simulink model "SIMULINK_ADP_Tracking"  (R2023b)
settings: Solver=FixedStepAuto  StartTime=0.0  StopTime=sim_end_time  FixedStep=fixed_step_size  RelTol=1e-3
undefined symbols (not defined in the file): a, act_end, b, battery_threshold, bb, delta_, draw_gif, droneyeeUAV2_NUM, droneyeeUAV3_NUM, droneyeeUAV4_NUM, droneyeeUAV5_NUM, fixed_step_size, k, KD_x, KD_y, kd_z, KDD_x, KDD_y, KI_x, KI_y, ki_z, KII_x, KII_y, KP_x, KP_y, kp_z, KPP_x, KPP_y, lmt, omega, omega_, R, sim_end_time, uav10num, uav1num, uav2num, uav3num, uav4num, uav5num, uav6num, uav7num, uav8num, uav9num, UAV_NUM, Vel_Switch_1, Vel_Switch_10, Vel_Switch_11, Vel_Switch_12, Vel_Switch_13, Vel_Switch_14, Vel_Switch_15, Vel_Switch_16, Vel_Switch_17, Vel_Switch_18, Vel_Switch_19, Vel_Switch_2, Vel_Switch_20, Vel_Switch_3, Vel_Switch_4, Vel_Switch_5 ... (+16)
libraries: simulink x118, aerolibanimutils x1
(part 3 of 11)

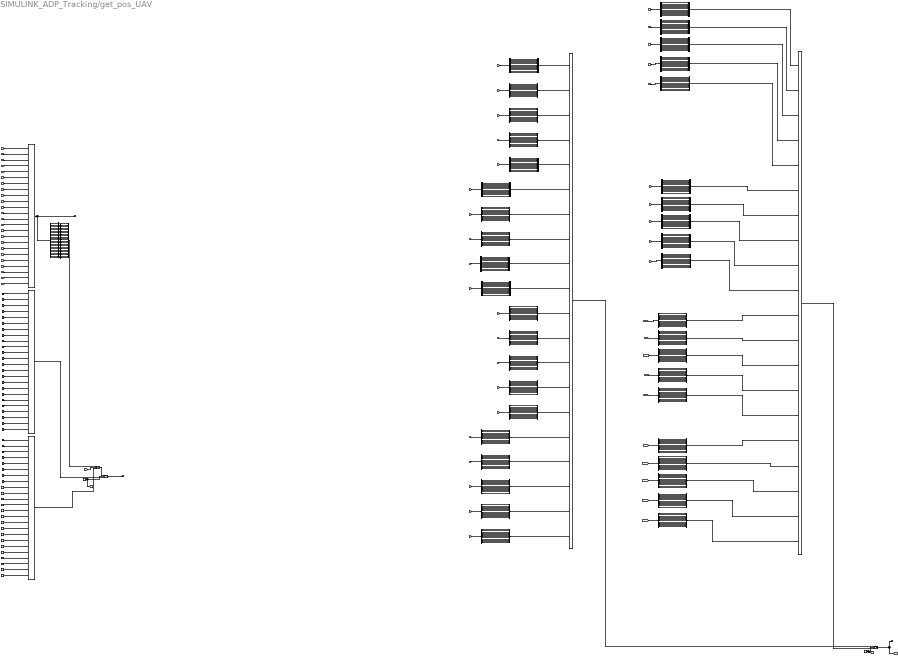
== system SIMULINK_ADP_Tracking/get_pos_UAV ==
  Bus Creator{1..20,37..42,46..49,51..60} (40 alike) : BusCreator  Inputs=12
  Bus Creator{34..36,62} (4 alike) : BusCreator  Inputs=24
  Bus Creator50 : BusCreator  Inputs=20
  Bus Creator61 : BusCreator  Inputs=20
  Bus Selector : BusSelector  OutputSignals=droneyeeUAV1bat,droneyeeUAV2bat,droneyeeUAV3bat,droneyeeUAV4bat,droneyeeUAV5bat,droneyeeUAV6bat,droneyeeUAV7bat,droneyeeUAV8bat,droneyeeUAV9bat,droneyeeUAV10bat,droneyeeUAV11bat,droneyeeUAV12bat,droneyeeUAV13bat,droneyeeUAV14bat,droneyeeUAV15bat,droneyeeUAV16bat,droneyeeUAV17bat,droneyeeUAV18bat,droneyeeUAV19bat,droneyeeUAV20bat,droneyeeUAV21bat,droneyeeUAV22bat,droneyeeUAV23bat,droneyeeUAV24bat
  Constant{,1..24} (25 alike) : Constant  Value=-1
  Constant25 : Constant
  Constant{26..49} (24 alike) : Constant  Value=100
  Demux{,16..23,40..41,52..57,59..62,66,68..69} (24 alike) : Demux  Outputs=3
  Demux{1..15,24..29,70..71,74..90} (40 alike) : Demux  Outputs=12
  Switch : Switch  SaturateOnIntegerOverflow=off  InputSameDT=off
  Switch1 : Switch  Criteria=u2 > Threshold  OutDataTypeStr=Inherit: Inherit via back propagation  SaturateOnIntegerOverflow=off  InputSameDT=off
  Switch2 : Switch  Criteria=u2 > Threshold  OutDataTypeStr=Inherit: Inherit via back propagation  SaturateOnIntegerOverflow=off  InputSameDT=off
  droneyeeUAV_batDIS : Outport  VectorParamsAs1DForOutWhenUnconnected=off
  droneyeeUAVbat1 : Outport  Port=2  VectorParamsAs1DForOutWhenUnconnected=off
  states1 : Outport  Port=3  VectorParamsAs1DForOutWhenUnconnected=off
  tag scope: sim_flag=global, switch_flag=global, uav_states=global
  wires:
  [battery_3] -> Bus Creator35/3  "droneyeeUAV3bat"
  [battery_1] -> Bus Creator35/1  "droneyeeUAV1bat"
  [battery_9] -> Bus Creator35/9  "droneyeeUAV9bat"
  [battery_2] -> Bus Creator35/2  "droneyeeUAV2bat"
  [battery_17] -> Bus Creator35/17  "droneyeeUAV17bat"
  [battery_6] -> Bus Creator35/6  "droneyeeUAV6bat"
  [battery_15] -> Bus Creator35/15  "droneyeeUAV15bat"
  [battery_12] -> Bus Creator35/12  "droneyeeUAV12bat"
  [battery_16] -> Bus Creator35/16  "droneyeeUAV16bat"
  [battery_11] -> Bus Creator35/11  "droneyeeUAV11bat"
  [battery_13] -> Bus Creator35/13  "droneyeeUAV13bat"
  [battery_19] -> Bus Creator35/19  "droneyeeUAV19bat"
  [battery_14] -> Bus Creator35/14  "droneyeeUAV14bat"
  [battery_20] -> Bus Creator35/20  "droneyeeUAV20bat"
  [battery_10] -> Bus Creator35/10  "droneyeeUAV10bat"
  Bus Creator35/1 -> Bus Selector/1, droneyeeUAV_batDIS/1
  [battery_18] -> Bus Creator35/18  "droneyeeUAV18bat"
  [battery_7] -> Bus Creator35/7  "droneyeeUAV7bat"
  [battery_8] -> Bus Creator35/8  "droneyeeUAV8bat"
  [battery_4] -> Bus Creator35/4  "droneyeeUAV4bat"
  [battery_23] -> Bus Creator35/23  "droneyeeUAV23bat"
  [battery_22] -> Bus Creator35/22  "droneyeeUAV22bat"
  [battery_21] -> Bus Creator35/21  "droneyeeUAV21bat"
  [battery_24] -> Bus Creator35/24  "droneyeeUAV24bat"
  [battery_5] -> Bus Creator35/5  "droneyeeUAV5bat"
  Constant1/1 -> Bus Creator34/2  "droneyeeUAV2bat"
  Constant4/1 -> Bus Creator34/5  "droneyeeUAV5bat"
  Constant18/1 -> Bus Creator34/19  "droneyeeUAV19bat"
  Constant20/1 -> Bus Creator34/21  "droneyeeUAV21bat"
  Constant2/1 -> Bus Creator34/3  "droneyeeUAV3bat"
  Bus Creator34/1 -> Switch/3
  Constant23/1 -> Bus Creator34/24  "droneyeeUAV24bat"
  Constant6/1 -> Bus Creator34/7  "droneyeeUAV7bat"
  Constant15/1 -> Bus Creator34/16  "droneyeeUAV16bat"
  Constant9/1 -> Bus Creator34/10  "droneyeeUAV10bat"
  Constant5/1 -> Bus Creator34/6  "droneyeeUAV6bat"
  Constant14/1 -> Bus Creator34/15  "droneyeeUAV15bat"
  Constant17/1 -> Bus Creator34/18  "droneyeeUAV18bat"
  Constant22/1 -> Bus Creator34/23  "droneyeeUAV23bat"
  Constant8/1 -> Bus Creator34/9  "droneyeeUAV9bat"
  Constant7/1 -> Bus Creator34/8  "droneyeeUAV8bat"
  Constant10/1 -> Bus Creator34/11  "droneyeeUAV11bat"
  Constant21/1 -> Bus Creator34/22  "droneyeeUAV22bat"
  Constant11/1 -> Bus Creator34/12  "droneyeeUAV12bat"
  Constant13/1 -> Bus Creator34/14  "droneyeeUAV14bat"
  Constant19/1 -> Bus Creator34/20  "droneyeeUAV20bat"
  Constant16/1 -> Bus Creator34/17  "droneyeeUAV17bat"
  Constant12/1 -> Bus Creator34/13  "droneyeeUAV13bat"
  Constant/1 -> Bus Creator34/1  "droneyeeUAV1bat"
  Constant3/1 -> Bus Creator34/4  "droneyeeUAV4bat"
  Bus Selector/1 -> Demux/1  "<droneyeeUAV1bat>"
  Demux/2 -> Bus Creator36/1  "droneyeeUAV1bat"
  Demux16/2 -> Bus Creator36/2  "droneyeeUAV2bat"
  Bus Selector/2 -> Demux16/1  "<droneyeeUAV2bat>"
  Bus Selector/3 -> Demux17/1  "<droneyeeUAV3bat>"
  Demux17/2 -> Bus Creator36/3  "droneyeeUAV3bat"
  Demux18/2 -> Bus Creator36/4  "droneyeeUAV4bat"
  Bus Selector/4 -> Demux18/1  "<droneyeeUAV4bat>"
  Bus Selector/5 -> Demux19/1  "<droneyeeUAV5bat>"
  Demux19/2 -> Bus Creator36/5  "droneyeeUAV5bat"
  Demux20/2 -> Bus Creator36/6  "droneyeeUAV6bat"
  Bus Selector/6 -> Demux20/1  "<droneyeeUAV6bat>"
  Bus Selector/7 -> Demux21/1  "<droneyeeUAV7bat>"
  Bus Selector/8 -> Demux22/1  "<droneyeeUAV8bat>"
  Bus Selector/9 -> Demux23/1  "<droneyeeUAV9bat>"
  Bus Selector/10 -> Demux40/1  "<droneyeeUAV10bat>"
  Bus Selector/11 -> Demux41/1  "<droneyeeUAV11bat>"
  Demux21/2 -> Bus Creator36/7  "droneyeeUAV7bat"
  Demux22/2 -> Bus Creator36/8  "droneyeeUAV8bat"
  Demux23/2 -> Bus Creator36/9  "droneyeeUAV9bat"
  Demux40/2 -> Bus Creator36/10  "droneyeeUAV10bat"
  Demux41/2 -> Bus Creator36/11  "droneyeeUAV11bat"
  Bus Selector/12 -> Demux52/1  "<droneyeeUAV12bat>"
  Demux52/2 -> Bus Creator36/12  "droneyeeUAV12bat"
  Bus Selector/13 -> Demux53/1  "<droneyeeUAV13bat>"
  Demux53/2 -> Bus Creator36/13  "droneyeeUAV13bat"
  Bus Selector/14 -> Demux54/1  "<droneyeeUAV14bat>"
  Demux54/2 -> Bus Creator36/14  "droneyeeUAV14bat"
  Bus Selector/15 -> Demux55/1  "<droneyeeUAV15bat>"
  Demux56/2 -> Bus Creator36/16  "droneyeeUAV16bat"
  Bus Selector/17 -> Demux57/1  "<droneyeeUAV17bat>"
  Demux59/2 -> Bus Creator36/18  "droneyeeUAV18bat"
  Demux55/2 -> Bus Creator36/15  "droneyeeUAV15bat"
  Bus Selector/16 -> Demux56/1  "<droneyeeUAV16bat>"
  Demux57/2 -> Bus Creator36/17  "droneyeeUAV17bat"
  Bus Selector/18 -> Demux59/1  "<droneyeeUAV18bat>"
  Bus Selector/19 -> Demux60/1  "<droneyeeUAV19bat>"
  Bus Selector/20 -> Demux61/1  "<droneyeeUAV20bat>"
  Demux61/2 -> Bus Creator36/20  "droneyeeUAV20bat"
  Demux60/2 -> Bus Creator36/19  "droneyeeUAV19bat"
  Bus Selector/21 -> Demux62/1  "<droneyeeUAV21bat>"
  Demux62/2 -> Bus Creator36/21  "droneyeeUAV21bat"
  Demux66/2 -> Bus Creator36/22  "droneyeeUAV22bat"
  Bus Selector/22 -> Demux66/1  "<droneyeeUAV22bat>"
  Bus Selector/23 -> Demux68/1  "<droneyeeUAV23bat>"
  Demux68/2 -> Bus Creator36/23  "droneyeeUAV23bat"
  Demux69/2 -> Bus Creator36/24  "droneyeeUAV24bat"
  Bus Selector/24 -> Demux69/1  "<droneyeeUAV24bat>"
  Bus Creator36/1 -> Switch2/1
  Constant24/1 -> Switch/2, [switch_flag]
  Switch/1 -> droneyeeUAVbat1/1
  [copterRev5] -> Demux9/1
  Bus Creator37/1 -> Bus Creator50/5  "droneyeeUAV5_states"
  [copterRev4] -> Demux70/1
  [copterRev3] -> Demux71/1
  [copterRev2] -> Demux74/1
  [copterRev1] -> Demux75/1
  [copterRev12] -> Demux78/1
  [copterRev14] -> Demux76/1
  [copterRev11] -> Demux79/1
  [copterRev15] -> Demux80/1
  [copterRev13] -> Demux77/1
  Bus Creator42/1 -> Bus Creator50/15  "droneyeeCAR5_states"
  Bus Creator41/1 -> Bus Creator50/1  "droneyeeUAV1_states"
  Bus Creator40/1 -> Bus Creator50/2  "droneyeeUAV2_states"
  Bus Creator39/1 -> Bus Creator50/3  "droneyeeUAV3_states"
  Bus Creator38/1 -> Bus Creator50/4  "droneyeeUAV4_states"
  Bus Creator49/1 -> Bus Creator50/11  "droneyeeCAR1_states"
  Bus Creator48/1 -> Bus Creator50/12  "droneyeeCAR2_states"
  Bus Creator47/1 -> Bus Creator50/13  "droneyeeCAR3_states"
  Bus Creator46/1 -> Bus Creator50/14  "droneyeeCAR4_states"
  Switch1/1 -> [uav_states], states1/1  "states"
  Demux75/4 -> Bus Creator41/4  "roll"
  Demux75/1 -> Bus Creator41/1  "x"
  Demux75/5 -> Bus Creator41/5  "pitch"
  Demux75/2 -> Bus Creator41/2  "y"
  Demux75/7 -> Bus Creator41/7  "latitude(degE7)"
  Demux75/8 -> Bus Creator41/8  "longitude\t(degE7)"
  Demux75/3 -> Bus Creator41/3  "z"
  Demux75/6 -> Bus Creator41/6  "yaw"
  Demux75/9 -> Bus Creator41/9  "alttude(mm)"
  Demux75/10 -> Bus Creator41/10  "x(home position)"
  Demux75/11 -> Bus Creator41/11  "y(home position)"
  Demux75/12 -> Bus Creator41/12  "z(home position)"
  Demux79/1 -> Bus Creator49/1  "x"
  Demux79/12 -> Bus Creator49/12  "z(home position)"
  Demux79/4 -> Bus Creator49/4  "roll"
  Demux79/3 -> Bus Creator49/3  "z"
  Demux79/8 -> Bus Creator49/8  "longitude\t(degE7)"
  Demux79/2 -> Bus Creator49/2  "y"
  Demux79/10 -> Bus Creator49/10  "x(home position)"
  Demux79/5 -> Bus Creator49/5  "pitch"
  Demux79/9 -> Bus Creator49/9  "alttude(mm)"
  Demux79/7 -> Bus Creator49/7  "latitude(degE7)"
  Demux79/6 -> Bus Creator49/6  "yaw"
  Demux79/11 -> Bus Creator49/11  "y(home position)"
  Demux78/1 -> Bus Creator48/1  "x"
  Demux78/12 -> Bus Creator48/12  "z(home position)"
  Demux78/4 -> Bus Creator48/4  "roll"
  Demux78/3 -> Bus Creator48/3  "z"
  Demux78/8 -> Bus Creator48/8  "longitude\t(degE7)"
  Demux78/2 -> Bus Creator48/2  "y"
  Demux78/10 -> Bus Creator48/10  "x(home position)"
  Demux78/5 -> Bus Creator48/5  "pitch"
  Demux78/9 -> Bus Creator48/9  "alttude(mm)"
  Demux78/7 -> Bus Creator48/7  "latitude(degE7)"
  Demux78/6 -> Bus Creator48/6  "yaw"
  Demux78/11 -> Bus Creator48/11  "y(home position)"
  Demux77/1 -> Bus Creator47/1  "x"
  Demux77/12 -> Bus Creator47/12  "z(home position)"
  Demux77/4 -> Bus Creator47/4  "roll"
  Demux77/3 -> Bus Creator47/3  "z"
  Demux77/8 -> Bus Creator47/8  "longitude\t(degE7)"
  Demux77/2 -> Bus Creator47/2  "y"
  Demux77/10 -> Bus Creator47/10  "x(home position)"
  Demux77/5 -> Bus Creator47/5  "pitch"
  Demux77/9 -> Bus Creator47/9  "alttude(mm)"
  Demux77/7 -> Bus Creator47/7  "latitude(degE7)"
  Demux77/6 -> Bus Creator47/6  "yaw"
  Demux77/11 -> Bus Creator47/11  "y(home position)"
  Demux76/1 -> Bus Creator46/1  "x"
  Demux76/12 -> Bus Creator46/12  "z(home position)"
  Demux76/4 -> Bus Creator46/4  "roll"
  Demux76/3 -> Bus Creator46/3  "z"
  Demux76/8 -> Bus Creator46/8  "longitude\t(degE7)"
  Demux76/2 -> Bus Creator46/2  "y"
  Demux76/10 -> Bus Creator46/10  "x(home position)"
  Demux76/5 -> Bus Creator46/5  "pitch"
  Demux76/9 -> Bus Creator46/9  "alttude(mm)"
  Demux76/7 -> Bus Creator46/7  "latitude(degE7)"
  Demux76/6 -> Bus Creator46/6  "yaw"
  Demux76/11 -> Bus Creator46/11  "y(home position)"
  Demux80/1 -> Bus Creator42/1  "x"
  Demux80/12 -> Bus Creator42/12  "z(home position)"
  Demux80/4 -> Bus Creator42/4  "roll"
  Demux80/3 -> Bus Creator42/3  "z"
  Demux80/8 -> Bus Creator42/8  "longitude\t(degE7)"
  Demux80/2 -> Bus Creator42/2  "y"
  Demux80/10 -> Bus Creator42/10  "x(home position)"
  Demux80/5 -> Bus Creator42/5  "pitch"
  Demux80/9 -> Bus Creator42/9  "alttude(mm)"
  Demux80/7 -> Bus Creator42/7  "latitude(degE7)"
  Demux80/6 -> Bus Creator42/6  "yaw"
  Demux80/11 -> Bus Creator42/11  "y(home position)"
  Demux74/10 -> Bus Creator40/10  "x(home position)"
  Demux74/12 -> Bus Creator40/12  "z(home position)"
  Demux74/7 -> Bus Creator40/7  "latitude(degE7)"
  Demux74/8 -> Bus Creator40/8  "longitude\t(degE7)"
  Demux74/9 -> Bus Creator40/9  "alttude(mm)"
  Demux74/1 -> Bus Creator40/1  "x"
  Demux74/2 -> Bus Creator40/2  "y"
  Demux74/3 -> Bus Creator40/3  "z"
  Demux74/4 -> Bus Creator40/4  "roll"
  Demux74/5 -> Bus Creator40/5  "pitch"
  Demux74/6 -> Bus Creator40/6  "yaw"
  Demux74/11 -> Bus Creator40/11  "y(home position)"
  Demux71/10 -> Bus Creator39/10  "x(home position)"
  Demux71/12 -> Bus Creator39/12  "z(home position)"
  Demux71/7 -> Bus Creator39/7  "latitude(degE7)"
  Demux71/8 -> Bus Creator39/8  "longitude\t(degE7)"
  Demux71/9 -> Bus Creator39/9  "alttude(mm)"
  Demux71/1 -> Bus Creator39/1  "x"
  Demux71/2 -> Bus Creator39/2  "y"
  Demux71/3 -> Bus Creator39/3  "z"
  Demux71/4 -> Bus Creator39/4  "roll"
  Demux71/5 -> Bus Creator39/5  "pitch"
  Demux71/6 -> Bus Creator39/6  "yaw"
  Demux71/11 -> Bus Creator39/11  "y(home position)"
  Demux70/10 -> Bus Creator38/10  "x(home position)"
  Demux70/12 -> Bus Creator38/12  "z(home position)"
  Demux70/7 -> Bus Creator38/7  "latitude(degE7)"
  Demux70/8 -> Bus Creator38/8  "longitude\t(degE7)"
  Demux70/9 -> Bus Creator38/9  "alttude(mm)"
  Demux70/1 -> Bus Creator38/1  "x"
  Demux70/2 -> Bus Creator38/2  "y"
  Demux70/3 -> Bus Creator38/3  "z"
  Demux70/4 -> Bus Creator38/4  "roll"
  Demux70/5 -> Bus Creator38/5  "pitch"
  Demux70/6 -> Bus Creator38/6  "yaw"
  Demux70/11 -> Bus Creator38/11  "y(home position)"
  Demux9/10 -> Bus Creator37/10  "x(home position)"
  Demux9/12 -> Bus Creator37/12  "z(home position)"
  Demux9/7 -> Bus Creator37/7  "latitude(degE7)"
  Demux9/8 -> Bus Creator37/8  "longitude\t(degE7)"
  Demux9/9 -> Bus Creator37/9  "alttude(mm)"
  Demux9/1 -> Bus Creator37/1  "x"
  Demux9/2 -> Bus Creator37/2  "y"
  Demux9/3 -> Bus Creator37/3  "z"
  Demux9/4 -> Bus Creator37/4  "roll"
  Demux9/5 -> Bus Creator37/5  "pitch"
  Demux9/6 -> Bus Creator37/6  "yaw"
  Demux9/11 -> Bus Creator37/11  "y(home position)"
  Constant25/1 -> [sim_flag], Switch1/2
  Demux87/6 -> Bus Creator59/6  "yaw"
  Demux90/6 -> Bus Creator51/6  "yaw"
  Demux85/3 -> Bus Creator57/3  "z"
  Demux89/1 -> Bus Creator56/1  "x"
  Demux81/2 -> Bus Creator52/2  "y"
  Demux87/7 -> Bus Creator59/7  "latitude(degE7)"
  Demux90/10 -> Bus Creator51/10  "x(home position)"
  Demux85/7 -> Bus Creator57/7  "latitude(degE7)"
  Demux82/9 -> Bus Creator53/9  "alttude(mm)"
  Demux82/12 -> Bus Creator53/12  "z(home position)"
  Demux90/11 -> Bus Creator51/11  "y(home position)"
  Demux90/4 -> Bus Creator51/4  "roll"
  Demux85/1 -> Bus Creator57/1  "x"
  Demux89/6 -> Bus Creator56/6  "yaw"
  Demux87/1 -> Bus Creator59/1  "x"
  Demux90/3 -> Bus Creator51/3  "z"
  Demux90/2 -> Bus Creator51/2  "y"
  Demux90/8 -> Bus Creator51/8  "longitude\t(degE7)"
  Demux85/6 -> Bus Creator57/6  "yaw"
  Demux81/11 -> Bus Creator52/11  "y(home position)"
  Demux81/9 -> Bus Creator52/9  "alttude(mm)"
  Demux82/7 -> Bus Creator53/7  "latitude(degE7)"
  Demux82/1 -> Bus Creator53/1  "x"
  Demux83/9 -> Bus Creator54/9  "alttude(mm)"
  Demux83/1 -> Bus Creator54/1  "x"
  Demux85/9 -> Bus Creator57/9  "alttude(mm)"
  Demux81/7 -> Bus Creator52/7  "latitude(degE7)"
  Demux81/10 -> Bus Creator52/10  "x(home position)"
  Demux83/6 -> Bus Creator54/6  "yaw"
  Demux81/12 -> Bus Creator52/12  "z(home position)"
  Bus Creator51/1 -> Bus Creator61/5  "droneyeeUAV5_states"
  Demux83/4 -> Bus Creator54/4  "roll"
  Demux81/8 -> Bus Creator52/8  "longitude\t(degE7)"
  Demux82/10 -> Bus Creator53/10  "x(home position)"
  Demux88/4 -> Bus Creator60/4  "roll"
  Demux90/5 -> Bus Creator51/5  "pitch"
  Demux89/10 -> Bus Creator56/10  "x(home position)"
  Demux86/11 -> Bus Creator58/11  "y(home position)"
  Demux89/4 -> Bus Creator56/4  "roll"
  Demux83/2 -> Bus Creator54/2  "y"
  Demux88/6 -> Bus Creator60/6  "yaw"
  Demux82/4 -> Bus Creator53/4  "roll"
  Demux90/7 -> Bus Creator51/7  "latitude(degE7)"
  Demux89/11 -> Bus Creator56/11  "y(home position)"
  Demux81/3 -> Bus Creator52/3  "z"
  Demux81/6 -> Bus Creator52/6  "yaw"
  Demux86/3 -> Bus Creator58/3  "z"
  Demux86/1 -> Bus Creator58/1  "x"
  Demux85/11 -> Bus Creator57/11  "y(home position)"
  Demux89/8 -> Bus Creator56/8  "longitude\t(degE7)"
  Demux81/1 -> Bus Creator52/1  "x"
  Demux86/6 -> Bus Creator58/6  "yaw"
  Demux83/7 -> Bus Creator54/7  "latitude(degE7)"
  [sim_CopterRec3] -> Demux82/1
  Demux82/3 -> Bus Creator53/3  "z"
  Demux85/2 -> Bus Creator57/2  "y"
  Demux82/11 -> Bus Creator53/11  "y(home position)"
  Demux83/3 -> Bus Creator54/3  "z"
  Demux87/9 -> Bus Creator59/9  "alttude(mm)"
  Demux82/6 -> Bus Creator53/6  "yaw"
  Demux81/4 -> Bus Creator52/4  "roll"
  Demux88/2 -> Bus Creator60/2  "y"
  Demux86/4 -> Bus Creator58/4  "roll"
  Bus Creator55/1 -> Bus Creator61/1  "droneyeeUAV1_states"
  Demux87/2 -> Bus Creator59/2  "y"
  Bus Creator60/1 -> Bus Creator61/11  "droneyeeCAR1_states"
  Demux90/12 -> Bus Creator51/12  "z(home position)"
  Demux83/12 -> Bus Creator54/12  "z(home position)"
  Demux82/8 -> Bus Creator53/8  "longitude\t(degE7)"
  Demux85/12 -> Bus Creator57/12  "z(home position)"
  Demux85/10 -> Bus Creator57/10  "x(home position)"
  Demux86/8 -> Bus Creator58/8  "longitude\t(degE7)"
  Demux85/4 -> Bus Creator57/4  "roll"
  Demux90/1 -> Bus Creator51/1  "x"
  Demux86/9 -> Bus Creator58/9  "alttude(mm)"
  Demux83/11 -> Bus Creator54/11  "y(home position)"
  Demux82/5 -> Bus Creator53/5  "pitch"
  Bus Creator52/1 -> Bus Creator61/4  "droneyeeUAV4_states"
  Demux86/5 -> Bus Creator58/5  "pitch"
  Demux87/5 -> Bus Creator59/5  "pitch"
  Demux89/5 -> Bus Creator56/5  "pitch"
  Bus Creator54/1 -> Bus Creator61/2  "droneyeeUAV2_states"
  Demux87/11 -> Bus Creator59/11  "y(home position)"
  Demux87/12 -> Bus Creator59/12  "z(home position)"
  Demux89/2 -> Bus Creator56/2  "y"
  Demux88/12 -> Bus Creator60/12  "z(home position)"
  Demux86/7 -> Bus Creator58/7  "latitude(degE7)"
  Demux88/11 -> Bus Creator60/11  "y(home position)"
  Demux88/10 -> Bus Creator60/10  "x(home position)"
  Demux87/3 -> Bus Creator59/3  "z"
  Demux88/8 -> Bus Creator60/8  "longitude\t(degE7)"
  Demux81/5 -> Bus Creator52/5  "pitch"
  Demux88/1 -> Bus Creator60/1  "x"
  Demux85/8 -> Bus Creator57/8  "longitude\t(degE7)"
  Demux86/10 -> Bus Creator58/10  "x(home position)"
  Demux85/5 -> Bus Creator57/5  "pitch"
  Demux86/2 -> Bus Creator58/2  "y"
  Demux87/4 -> Bus Creator59/4  "roll"
  Demux86/12 -> Bus Creator58/12  "z(home position)"
  Demux89/9 -> Bus Creator56/9  "alttude(mm)"
  Demux87/10 -> Bus Creator59/10  "x(home position)"
  Bus Creator57/1 -> Bus Creator61/14  "droneyeeCAR4_states"
  Demux90/9 -> Bus Creator51/9  "alttude(mm)"
  Demux89/3 -> Bus Creator56/3  "z"
  Bus Creator58/1 -> Bus Creator61/13  "droneyeeCAR3_states"
  Bus Creator59/1 -> Bus Creator61/12  "droneyeeCAR2_states"
  [sim_CopterRec1] -> Demux84/1
  Demux88/3 -> Bus Creator60/3  "z"
  [sim_CopterRec4] -> Demux81/1
  Demux89/7 -> Bus Creator56/7  "latitude(degE7)"
  Bus Creator56/1 -> Bus Creator61/15  "droneyeeCAR5_states"
  Demux88/9 -> Bus Creator60/9  "alttude(mm)"
  Demux87/8 -> Bus Creator59/8  "longitude\t(degE7)"
  [sim_CopterRec2] -> Demux83/1
  Demux89/12 -> Bus Creator56/12  "z(home position)"
  Demux88/5 -> Bus Creator60/5  "pitch"
  Demux88/7 -> Bus Creator60/7  "latitude(degE7)"
  [sim_CopterRec5] -> Demux90/1
  Bus Creator53/1 -> Bus Creator61/3  "droneyeeUAV3_states"
  Demux82/2 -> Bus Creator53/2  "y"
  Demux83/8 -> Bus Creator54/8  "longitude\t(degE7)"
  Demux83/10 -> Bus Creator54/10  "x(home position)"
  Demux83/5 -> Bus Creator54/5  "pitch"
  Bus Creator61/1 -> Switch1/3
  [sim_flag] -> Switch2/2
  Switch2/1 -> Switch/1
  Constant39/1 -> Bus Creator62/21  "droneyeeUAV21bat"
  Constant37/1 -> Bus Creator62/20  "droneyeeUAV20bat"
  Constant44/1 -> Bus Creator62/5  "droneyeeUAV5bat"
  Constant35/1 -> Bus Creator62/18  "droneyeeUAV18bat"
  Constant27/1 -> Bus Creator62/2  "droneyeeUAV2bat"
  Constant43/1 -> Bus Creator62/4  "droneyeeUAV4bat"
  Constant33/1 -> Bus Creator62/14  "droneyeeUAV14bat"
  Constant31/1 -> Bus Creator62/12  "droneyeeUAV12bat"
  Constant32/1 -> Bus Creator62/13  "droneyeeUAV13bat"
  Constant29/1 -> Bus Creator62/10  "droneyeeUAV10bat"
  Constant42/1 -> Bus Creator62/24  "droneyeeUAV24bat"
  Constant26/1 -> Bus Creator62/1  "droneyeeUAV1bat"
  Constant34/1 -> Bus Creator62/17  "droneyeeUAV17bat"
  Constant38/1 -> Bus Creator62/3  "droneyeeUAV3bat"
  Constant47/1 -> Bus Creator62/8  "droneyeeUAV8bat"
  Constant46/1 -> Bus Creator62/7  "droneyeeUAV7bat"
  Constant48/1 -> Bus Creator62/15  "droneyeeUAV15bat"
  Constant41/1 -> Bus Creator62/23  "droneyeeUAV23bat"
  Constant36/1 -> Bus Creator62/19  "droneyeeUAV19bat"
  Constant28/1 -> Bus Creator62/9  "droneyeeUAV9bat"
  Constant45/1 -> Bus Creator62/6  "droneyeeUAV6bat"
  Constant40/1 -> Bus Creator62/22  "droneyeeUAV22bat"
  Constant49/1 -> Bus Creator62/16  "droneyeeUAV16bat"
  Constant30/1 -> Bus Creator62/11  "droneyeeUAV11bat"
  Bus Creator62/1 -> Switch2/3
  Demux84/7 -> Bus Creator55/7  "latitude(degE7)"
  Demux84/3 -> Bus Creator55/3  "z"
  Demux84/4 -> Bus Creator55/4  "roll"
  Demux84/2 -> Bus Creator55/2  "y"
  Demux84/9 -> Bus Creator55/9  "alttude(mm)"
  Demux84/10 -> Bus Creator55/10  "x(home position)"
  Demux84/12 -> Bus Creator55/12  "z(home position)"
  Demux84/5 -> Bus Creator55/5  "pitch"
  Demux84/6 -> Bus Creator55/6  "yaw"
  Demux84/1 -> Bus Creator55/1  "x"
  Demux84/8 -> Bus Creator55/8  "longitude\t(degE7)"
  Demux84/11 -> Bus Creator55/11  "y(home position)"
  Demux1/2 -> Bus Creator2/2  "y"
  Demux1/9 -> Bus Creator2/9  "alttude(mm)"
  Demux2/4 -> Bus Creator3/4  "roll"
  Demux3/8 -> Bus Creator4/8  "longitude\t(degE7)"
  Demux3/5 -> Bus Creator4/5  "pitch"
  Demux3/12 -> Bus Creator4/12  "z(home position)"
  Demux2/11 -> Bus Creator3/11  "y(home position)"
  Demux3/9 -> Bus Creator4/9  "alttude(mm)"
  Demux5/5 -> Bus Creator1/5  "pitch"
  Demux5/6 -> Bus Creator1/6  "yaw"
  Demux2/6 -> Bus Creator3/6  "yaw"
  Demux1/10 -> Bus Creator2/10  "x(home position)"
  Demux2/8 -> Bus Creator3/8  "longitude\t(degE7)"
  Demux5/4 -> Bus Creator1/4  "roll"
  Demux3/3 -> Bus Creator4/3  "z"
  Demux3/7 -> Bus Creator4/7  "latitude(degE7)"
  Demux4/10 -> Bus Creator5/10  "x(home position)"
  Demux2/5 -> Bus Creator3/5  "pitch"
  Demux4/5 -> Bus Creator5/5  "pitch"
  Demux3/10 -> Bus Creator4/10  "x(home position)"
  Demux2/10 -> Bus Creator3/10  "x(home position)"
  Demux3/2 -> Bus Creator4/2  "y"
  Demux1/4 -> Bus Creator2/4  "roll"
  Demux1/12 -> Bus Creator2/12  "z(home position)"
  Demux2/9 -> Bus Creator3/9  "alttude(mm)"
  Demux4/4 -> Bus Creator5/4  "roll"
  Demux4/7 -> Bus Creator5/7  "latitude(degE7)"
  Demux4/6 -> Bus Creator5/6  "yaw"
  [copterRev9] -> Demux1/1
  Demux4/12 -> Bus Creator5/12  "z(home position)"
  Demux4/9 -> Bus Creator5/9  "alttude(mm)"
  [copterRev8] -> Demux2/1
  Demux1/3 -> Bus Creator2/3  "z"
  [copterRev10] -> Demux5/1
  Demux4/8 -> Bus Creator5/8  "longitude\t(degE7)"
  Demux5/9 -> Bus Creator1/9  "alttude(mm)"
  Demux5/3 -> Bus Creator1/3  "z"
  [copterRev6] -> Demux4/1
  Demux5/8 -> Bus Creator1/8  "longitude\t(degE7)"
  Demux2/2 -> Bus Creator3/2  "y"
  Demux4/1 -> Bus Creator5/1  "x"
  Demux1/8 -> Bus Creator2/8  "longitude\t(degE7)"
  Demux5/12 -> Bus Creator1/12  "z(home position)"
  [copterRev7] -> Demux3/1
  Demux2/3 -> Bus Creator3/3  "z"
  Demux2/7 -> Bus Creator3/7  "latitude(degE7)"
  Demux5/1 -> Bus Creator1/1  "x"
  Demux5/2 -> Bus Creator1/2  "y"
  Demux3/6 -> Bus Creator4/6  "yaw"
  Demux2/1 -> Bus Creator3/1  "x"
  Demux1/5 -> Bus Creator2/5  "pitch"
  Demux5/11 -> Bus Creator1/11  "y(home position)"
  Demux3/1 -> Bus Creator4/1  "x"
  Demux2/12 -> Bus Creator3/12  "z(home position)"
  Demux4/3 -> Bus Creator5/3  "z"
  Demux4/2 -> Bus Creator5/2  "y"
  Demux5/7 -> Bus Creator1/7  "latitude(degE7)"
  Demux3/4 -> Bus Creator4/4  "roll"
  Demux1/1 -> Bus Creator2/1  "x"
  Demux4/11 -> Bus Creator5/11  "y(home position)"
  Demux1/7 -> Bus Creator2/7  "latitude(degE7)"
  Demux5/10 -> Bus Creator1/10  "x(home position)"
  Demux3/11 -> Bus Creator4/11  "y(home position)"
  Demux1/6 -> Bus Creator2/6  "yaw"
  Demux1/11 -> Bus Creator2/11  "y(home position)"
  Bus Creator5/1 -> Bus Creator50/6  "droneyeeUAV6_states"
  Bus Creator4/1 -> Bus Creator50/7  "droneyeeUAV7_states"
  Bus Creator3/1 -> Bus Creator50/8  "droneyeeUAV8_states"
  Bus Creator2/1 -> Bus Creator50/9  "droneyeeUAV9_states"
  Bus Creator1/1 -> Bus Creator50/10  "droneyeeUAV10_states"
  Demux10/2 -> Bus Creator10/2  "y"
  Demux10/9 -> Bus Creator10/9  "alttude(mm)"
  Demux11/6 -> Bus Creator6/6  "yaw"
  Demux11/5 -> Bus Creator6/5  "pitch"
  Demux11/10 -> Bus Creator6/10  "x(home position)"
  Demux11/2 -> Bus Creator6/2  "y"
  Demux6/6 -> Bus Creator7/6  "yaw"
  Demux7/11 -> Bus Creator8/11  "y(home position)"
  Demux6/8 -> Bus Creator7/8  "longitude\t(degE7)"
  Demux7/7 -> Bus Creator8/7  "latitude(degE7)"
  Demux7/2 -> Bus Creator8/2  "y"
  Demux7/3 -> Bus Creator8/3  "z"
  Demux10/8 -> Bus Creator10/8  "longitude\t(degE7)"
  Demux8/9 -> Bus Creator9/9  "alttude(mm)"
  Demux8/5 -> Bus Creator9/5  "pitch"
  Demux10/1 -> Bus Creator10/1  "x"
  Demux8/8 -> Bus Creator9/8  "longitude\t(degE7)"
  Demux8/3 -> Bus Creator9/3  "z"
  Demux8/6 -> Bus Creator9/6  "yaw"
  Demux8/12 -> Bus Creator9/12  "z(home position)"
  Demux10/6 -> Bus Creator10/6  "yaw"
  Demux10/11 -> Bus Creator10/11  "y(home position)"
  Demux6/9 -> Bus Creator7/9  "alttude(mm)"
  Demux11/1 -> Bus Creator6/1  "x"
  Demux11/11 -> Bus Creator6/11  "y(home position)"
  Demux7/1 -> Bus Creator8/1  "x"
  Demux7/8 -> Bus Creator8/8  "longitude\t(degE7)"
  Demux10/3 -> Bus Creator10/3  "z"
  Demux10/12 -> Bus Creator10/12  "z(home position)"
  Demux11/3 -> Bus Creator6/3  "z"
  [copterRev16] -> Demux10/1
  Demux6/4 -> Bus Creator7/4  "roll"
  Demux6/3 -> Bus Creator7/3  "z"
  Demux8/1 -> Bus Creator9/1  "x"
  Demux6/1 -> Bus Creator7/1  "x"
  Demux8/7 -> Bus Creator9/7  "latitude(degE7)"
  Demux6/10 -> Bus Creator7/10  "x(home position)"
  Demux7/6 -> Bus Creator8/6  "yaw"
  Demux7/9 -> Bus Creator8/9  "alttude(mm)"
  Demux7/4 -> Bus Creator8/4  "roll"
  [copterRev20] -> Demux11/1
  Demux6/7 -> Bus Creator7/7  "latitude(degE7)"
  Demux8/11 -> Bus Creator9/11  "y(home position)"
  Demux8/2 -> Bus Creator9/2  "y"
  Demux7/5 -> Bus Creator8/5  "pitch"
  Demux6/5 -> Bus Creator7/5  "pitch"
  Demux7/10 -> Bus Creator8/10  "x(home position)"
  Demux10/10 -> Bus Creator10/10  "x(home position)"
  [copterRev17] -> Demux8/1
  [copterRev19] -> Demux6/1
  Demux11/12 -> Bus Creator6/12  "z(home position)"
  Demux6/2 -> Bus Creator7/2  "y"
  Demux8/10 -> Bus Creator9/10  "x(home position)"
  Demux10/7 -> Bus Creator10/7  "latitude(degE7)"
  Demux6/11 -> Bus Creator7/11  "y(home position)"
  Demux10/4 -> Bus Creator10/4  "roll"
  Demux10/5 -> Bus Creator10/5  "pitch"
  Demux7/12 -> Bus Creator8/12  "z(home position)"
  Demux11/4 -> Bus Creator6/4  "roll"
  Demux6/12 -> Bus Creator7/12  "z(home position)"
  Demux8/4 -> Bus Creator9/4  "roll"
  [copterRev18] -> Demux7/1
  Demux11/9 -> Bus Creator6/9  "alttude(mm)"
  Demux11/7 -> Bus Creator6/7  "latitude(degE7)"
  Demux11/8 -> Bus Creator6/8  "longitude\t(degE7)"
  Bus Creator10/1 -> Bus Creator50/16  "droneyeeCAR6_states"
  Bus Creator9/1 -> Bus Creator50/17  "droneyeeCAR7_states"
  Bus Creator8/1 -> Bus Creator50/18  "droneyeeCAR8_states"
  Bus Creator7/1 -> Bus Creator50/19  "droneyeeCAR9_states"
  Bus Creator6/1 -> Bus Creator50/20  "droneyeeCAR10_states"
  Demux13/11 -> Bus Creator13/11  "y(home position)"
  Demux13/6 -> Bus Creator13/6  "yaw"
  Demux12/4 -> Bus Creator12/4  "roll"
  Demux13/3 -> Bus Creator13/3  "z"
  Demux14/8 -> Bus Creator14/8  "longitude\t(degE7)"
  Demux14/5 -> Bus Creator14/5  "pitch"
  Demux14/7 -> Bus Creator14/7  "latitude(degE7)"
  Demux14/11 -> Bus Creator14/11  "y(home position)"
  Demux15/2 -> Bus Creator15/2  "y"
  Demux24/10 -> Bus Creator11/10  "x(home position)"
  Demux15/10 -> Bus Creator15/10  "x(home position)"
  Demux13/8 -> Bus Creator13/8  "longitude\t(degE7)"
  Demux15/4 -> Bus Creator15/4  "roll"
  Demux12/2 -> Bus Creator12/2  "y"
  Demux15/3 -> Bus Creator15/3  "z"
  Demux15/9 -> Bus Creator15/9  "alttude(mm)"
  Demux24/6 -> Bus Creator11/6  "yaw"
  Demux14/12 -> Bus Creator14/12  "z(home position)"
  Demux15/11 -> Bus Creator15/11  "y(home position)"
  Demux13/4 -> Bus Creator13/4  "roll"
  Demux15/5 -> Bus Creator15/5  "pitch"
  Demux15/1 -> Bus Creator15/1  "x"
  Demux12/9 -> Bus Creator12/9  "alttude(mm)"
  Demux15/6 -> Bus Creator15/6  "yaw"
  Demux24/12 -> Bus Creator11/12  "z(home position)"
  Demux15/12 -> Bus Creator15/12  "z(home position)"
  Demux12/12 -> Bus Creator12/12  "z(home position)"
  Demux12/6 -> Bus Creator12/6  "yaw"
  Demux24/8 -> Bus Creator11/8  "longitude\t(degE7)"
  Demux12/3 -> Bus Creator12/3  "z"
  Demux24/5 -> Bus Creator11/5  "pitch"
  Demux14/6 -> Bus Creator14/6  "yaw"
  Demux14/10 -> Bus Creator14/10  "x(home position)"
  Demux14/4 -> Bus Creator14/4  "roll"
  Demux13/10 -> Bus Creator13/10  "x(home position)"
  Demux12/8 -> Bus Creator12/8  "longitude\t(degE7)"
  Demux14/2 -> Bus Creator14/2  "y"
  Demux12/10 -> Bus Creator12/10  "x(home position)"
  Demux14/1 -> Bus Creator14/1  "x"
  Demux12/1 -> Bus Creator12/1  "x"
  Demux14/9 -> Bus Creator14/9  "alttude(mm)"
  Demux13/1 -> Bus Creator13/1  "x"
  Demux24/9 -> Bus Creator11/9  "alttude(mm)"
  Demux12/11 -> Bus Creator12/11  "y(home position)"
  Demux24/1 -> Bus Creator11/1  "x"
  Demux15/8 -> Bus Creator15/8  "longitude\t(degE7)"
  Demux12/7 -> Bus Creator12/7  "latitude(degE7)"
  Demux13/9 -> Bus Creator13/9  "alttude(mm)"
  Demux24/11 -> Bus Creator11/11  "y(home position)"
  Demux24/4 -> Bus Creator11/4  "roll"
  Demux13/2 -> Bus Creator13/2  "y"
  Demux14/3 -> Bus Creator14/3  "z"
  Demux13/7 -> Bus Creator13/7  "latitude(degE7)"
  Demux13/12 -> Bus Creator13/12  "z(home position)"
  Demux12/5 -> Bus Creator12/5  "pitch"
  Demux24/2 -> Bus Creator11/2  "y"
  Demux15/7 -> Bus Creator15/7  "latitude(degE7)"
  Demux24/3 -> Bus Creator11/3  "z"
  Demux13/5 -> Bus Creator13/5  "pitch"
  Demux24/7 -> Bus Creator11/7  "latitude(degE7)"
  Bus Creator15/1 -> Bus Creator61/6  "droneyeeUAV6_states"
  Bus Creator14/1 -> Bus Creator61/7  "droneyeeUAV7_states"
  Bus Creator13/1 -> Bus Creator61/8  "droneyeeUAV8_states"
  Bus Creator12/1 -> Bus Creator61/9  "droneyeeUAV9_states"
  Bus Creator11/1 -> Bus Creator61/10  "droneyeeUAV10_states"
  Bus Creator18/1 -> Bus Creator61/18  "droneyeeCAR8_states"
  Bus Creator19/1 -> Bus Creator61/17  "droneyeeCAR7_states"
  Demux28/3 -> Bus Creator20/3  "z"
  Demux27/4 -> Bus Creator19/4  "roll"
  Demux26/2 -> Bus Creator18/2  "y"
  [sim_CarRec8] -> Demux26/1
  Demux27/8 -> Bus Creator19/8  "longitude\t(degE7)"
  Demux27/1 -> Bus Creator19/1  "x"
  Demux26/12 -> Bus Creator18/12  "z(home position)"
  Demux29/9 -> Bus Creator16/9  "alttude(mm)"
  Demux26/3 -> Bus Creator18/3  "z"
  Demux27/10 -> Bus Creator19/10  "x(home position)"
  Demux26/7 -> Bus Creator18/7  "latitude(degE7)"
  Demux29/3 -> Bus Creator16/3  "z"
  [sim_CarRec9] -> Demux25/1
  Bus Creator16/1 -> Bus Creator61/20  "droneyeeCAR10_states"
  Demux25/11 -> Bus Creator17/11  "y(home position)"
  Demux25/5 -> Bus Creator17/5  "pitch"
  Demux26/9 -> Bus Creator18/9  "alttude(mm)"
  Demux28/12 -> Bus Creator20/12  "z(home position)"
  Demux25/6 -> Bus Creator17/6  "yaw"
  Demux29/12 -> Bus Creator16/12  "z(home position)"
  Demux26/1 -> Bus Creator18/1  "x"
  [sim_CarRec6] -> Demux28/1
  [sim_CarRec7] -> Demux27/1
  Demux29/10 -> Bus Creator16/10  "x(home position)"
  Demux29/7 -> Bus Creator16/7  "latitude(degE7)"
  Demux28/4 -> Bus Creator20/4  "roll"
  Demux29/8 -> Bus Creator16/8  "longitude\t(degE7)"
  Demux26/6 -> Bus Creator18/6  "yaw"
  Demux25/2 -> Bus Creator17/2  "y"
  Demux25/9 -> Bus Creator17/9  "alttude(mm)"
  Demux28/7 -> Bus Creator20/7  "latitude(degE7)"
  Demux29/2 -> Bus Creator16/2  "y"
  Demux27/12 -> Bus Creator19/12  "z(home position)"
  Demux29/6 -> Bus Creator16/6  "yaw"
  Demux29/5 -> Bus Creator16/5  "pitch"
  Demux26/5 -> Bus Creator18/5  "pitch"
  Demux28/6 -> Bus Creator20/6  "yaw"
  Demux29/4 -> Bus Creator16/4  "roll"
  Demux26/8 -> Bus Creator18/8  "longitude\t(degE7)"
  Demux25/10 -> Bus Creator17/10  "x(home position)"
  Demux25/4 -> Bus Creator17/4  "roll"
  Demux26/4 -> Bus Creator18/4  "roll"
  Demux28/2 -> Bus Creator20/2  "y"
  Demux27/11 -> Bus Creator19/11  "y(home position)"
  Demux27/5 -> Bus Creator19/5  "pitch"
  Demux27/6 -> Bus Creator19/6  "yaw"
  Demux25/7 -> Bus Creator17/7  "latitude(degE7)"
  Demux27/9 -> Bus Creator19/9  "alttude(mm)"
  Demux26/11 -> Bus Creator18/11  "y(home position)"
  Demux25/8 -> Bus Creator17/8  "longitude\t(degE7)"
  Demux27/2 -> Bus Creator19/2  "y"
  Demux28/1 -> Bus Creator20/1  "x"
  [sim_CarRec10] -> Demux29/1
  Demux27/7 -> Bus Creator19/7  "latitude(degE7)"
  Demux25/3 -> Bus Creator17/3  "z"
  Demux29/11 -> Bus Creator16/11  "y(home position)"
  Demux28/9 -> Bus Creator20/9  "alttude(mm)"
  Demux28/11 -> Bus Creator20/11  "y(home position)"
  Demux28/5 -> Bus Creator20/5  "pitch"
  Demux26/10 -> Bus Creator18/10  "x(home position)"
  Demux27/3 -> Bus Creator19/3  "z"
  Bus Creator17/1 -> Bus Creator61/19  "droneyeeCAR9_states"
  Demux28/10 -> Bus Creator20/10  "x(home position)"
  Demux29/1 -> Bus Creator16/1  "x"
  Bus Creator20/1 -> Bus Creator61/16  "droneyeeCAR6_states"
  Demux25/12 -> Bus Creator17/12  "z(home position)"
  Demux28/8 -> Bus Creator20/8  "longitude\t(degE7)"
  Demux25/1 -> Bus Creator17/1  "x"
  [sim_CopterRec6] -> Demux15/1
  [sim_CopterRec8] -> Demux13/1
  [sim_CopterRec7] -> Demux14/1
  [sim_CopterRec10] -> Demux24/1
  [sim_CopterRec9] -> Demux12/1
  [sim_CarRec5] -> Demux89/1
  [sim_CarRec3] -> Demux86/1
  [sim_CarRec2] -> Demux87/1
  [sim_CarRec4] -> Demux85/1
  [sim_CarRec1] -> Demux88/1
  Bus Creator50/1 -> Switch1/1  "states"

== system SIMULINK_ADP_Tracking/plot ==
  In1 : Inport
  Bus Selector : BusSelector  OutputSignals=droneyeeUAV1_2,droneyeeUAV3_4,droneyeeUAV5_6,droneyeeUAV7_8,droneyeeUAV9_10,uva11_12,uav13_14,uav15_16,uav17_18,uav19_20,uav21_22,uav23_24
  Bus Selector1 : BusSelector  OutputSignals=droneyeeUAV1_states.x1,droneyeeUAV1_states.y1,droneyeeUAV1_states.z1,droneyeeUAV2_states.x2,droneyeeUAV2_states.y2,droneyeeUAV2_states.z2
  Bus Selector10 : BusSelector  OutputSignals=droneyeeUAV17_states.x7,droneyeeUAV17_states.y7,droneyeeUAV17_states.z7,droneyeeUAV18_states.x8,droneyeeUAV18_states.y8,droneyeeUAV18_states.z8
  Bus Selector11 : BusSelector  OutputSignals=droneyeeUAV19_states.x9,droneyeeUAV19_states.y9,droneyeeUAV19_states.z9,droneyeeUAV20_states.x10,droneyeeUAV20_states.y10,droneyeeUAV20_states.z10
  Bus Selector12 : BusSelector  OutputSignals=droneyeeUAV23_states.x3,droneyeeUAV23_states.y3,droneyeeUAV23_states.z3,droneyeeUAV24_states.x4,droneyeeUAV24_states.y4,droneyeeUAV24_states.z4
  Bus Selector2 : BusSelector  OutputSignals=droneyeeUAV3_states.x3,droneyeeUAV3_states.y3,droneyeeUAV3_states.z3,droneyeeUAV4_states.x4,droneyeeUAV4_states.y4,droneyeeUAV4_states.z4
  Bus Selector3 : BusSelector  OutputSignals=droneyeeUAV5_states.x5,droneyeeUAV5_states.y5,droneyeeUAV5_states.z5,droneyeeUAV6_states.x6,droneyeeUAV6_states.y6,droneyeeUAV6_states.z6
  Bus Selector4 : BusSelector  OutputSignals=droneyeeUAV7_states.x7,droneyeeUAV7_states.y7,droneyeeUAV7_states.z7,droneyeeUAV8_states.x8,droneyeeUAV8_states.y8,droneyeeUAV8_states.z8
  Bus Selector5 : BusSelector  OutputSignals=droneyeeUAV9_states.x9,droneyeeUAV9_states.y9,droneyeeUAV9_states.z9,droneyeeUAV10_states.x10,droneyeeUAV10_states.y10,droneyeeUAV10_states.z10
  Bus Selector6 : BusSelector  OutputSignals=droneyeeUAV11_states.x1,droneyeeUAV11_states.y1,droneyeeUAV11_states.z1,droneyeeUAV12_states.x2,droneyeeUAV12_states.y2,droneyeeUAV12_states.z2
  Bus Selector7 : BusSelector  OutputSignals=droneyeeUAV13_states.x3,droneyeeUAV13_states.y3,droneyeeUAV13_states.z3,droneyeeUAV14_states.x4,droneyeeUAV14_states.y4,droneyeeUAV14_states.z4
  Bus Selector8 : BusSelector  OutputSignals=droneyeeUAV21_states.x1,droneyeeUAV21_states.y1,droneyeeUAV21_states.z1,droneyeeUAV22_states.x2,droneyeeUAV22_states.y2,droneyeeUAV22_states.z2
  Bus Selector9 : BusSelector  OutputSignals=droneyeeUAV15_states.x5,droneyeeUAV15_states.y5,droneyeeUAV15_states.z5,droneyeeUAV16_states.x6,droneyeeUAV16_states.y6,droneyeeUAV16_states.z6
  MATLAB Function : MATLAB Function  TreatAsAtomicUnit=on
  Subsystem : Subsystem
  wires:
  Subsystem/1(step_time) -> MATLAB Function/73(time_step)
  Subsystem/3(x_min) -> MATLAB Function/75(XMIN)
  Subsystem/4(x_max) -> MATLAB Function/76(XMAX)
  Subsystem/5(y_min) -> MATLAB Function/77(YMIN)
  Subsystem/6(y_max) -> MATLAB Function/78(YMAX)
  Subsystem/7(z_min) -> MATLAB Function/79(ZMIN)
  Subsystem/8(z_max) -> MATLAB Function/80(ZMAX)
  Subsystem/15(draw_gif) -> MATLAB Function/87(draw_gif)
  Subsystem/2(act_end) -> MATLAB Function/74(act_end)
  Subsystem/9(a) -> MATLAB Function/81(a)
  Subsystem/10(b) -> MATLAB Function/82(b)
  Subsystem/11(k) -> MATLAB Function/83(k)
  Subsystem/12(bb) -> MATLAB Function/84(bb)
  Subsystem/13(w1) -> MATLAB Function/85(w1)
  Subsystem/14(w2) -> MATLAB Function/86(w2)
  In1/1 -> Bus Selector/1
  Bus Selector/1 -> Bus Selector1/1  "<droneyeeUAV1_2>"
  Bus Selector1/1 -> MATLAB Function/1(x1)  "<x1>"
  Bus Selector1/2 -> MATLAB Function/2(y1)  "<y1>"
  Bus Selector1/3 -> MATLAB Function/3(z1)  "<z1>"
  Bus Selector1/4 -> MATLAB Function/4(x2)  "<x2>"
  Bus Selector1/5 -> MATLAB Function/5(y2)  "<y2>"
  Bus Selector1/6 -> MATLAB Function/6(z2)  "<z2>"
  Bus Selector/2 -> Bus Selector2/1  "<droneyeeUAV3_4>"
  Bus Selector2/1 -> MATLAB Function/7(x3)  "<x3>"
  Bus Selector2/2 -> MATLAB Function/8(y3)  "<y3>"
  Bus Selector2/3 -> MATLAB Function/9(z3)  "<z3>"
  Bus Selector2/4 -> MATLAB Function/10(x4)  "<x4>"
  Bus Selector2/5 -> MATLAB Function/11(y4)  "<y4>"
  Bus Selector2/6 -> MATLAB Function/12(z4)  "<z4>"
  Bus Selector3/1 -> MATLAB Function/13(x5)  "<x5>"
  Bus Selector3/2 -> MATLAB Function/14(y5)  "<y5>"
  Bus Selector3/3 -> MATLAB Function/15(z5)  "<z5>"
  Bus Selector3/4 -> MATLAB Function/16(x6)  "<x6>"
  Bus Selector3/5 -> MATLAB Function/17(y6)  "<y6>"
  Bus Selector3/6 -> MATLAB Function/18(z6)  "<z6>"
  Bus Selector/3 -> Bus Selector3/1  "<droneyeeUAV5_6>"
  Bus Selector4/1 -> MATLAB Function/19(x7)  "<x7>"
  Bus Selector4/2 -> MATLAB Function/20(y7)  "<y7>"
  Bus Selector4/3 -> MATLAB Function/21(z7)  "<z7>"
  Bus Selector4/4 -> MATLAB Function/22(x8)  "<x8>"
  Bus Selector4/5 -> MATLAB Function/23(y8)  "<y8>"
  Bus Selector4/6 -> MATLAB Function/24(z8)  "<z8>"
  Bus Selector/4 -> Bus Selector4/1  "<droneyeeUAV7_8>"
  Bus Selector5/1 -> MATLAB Function/25(x9)  "<x9>"
  Bus Selector5/2 -> MATLAB Function/26(y9)  "<y9>"
  Bus Selector5/3 -> MATLAB Function/27(z9)  "<z9>"
  Bus Selector5/4 -> MATLAB Function/28(x10)  "<x10>"
  Bus Selector5/5 -> MATLAB Function/29(y10)  "<y10>"
  Bus Selector5/6 -> MATLAB Function/30(z10)  "<z10>"
  Bus Selector/5 -> Bus Selector5/1  "<droneyeeUAV9_10>"
  Bus Selector6/1 -> MATLAB Function/31(x11)  "<x1>"
  Bus Selector6/2 -> MATLAB Function/32(y11)  "<y1>"
  Bus Selector6/3 -> MATLAB Function/33(z11)  "<z1>"
  Bus Selector6/4 -> MATLAB Function/34(x12)  "<x2>"
  Bus Selector6/5 -> MATLAB Function/35(y12)  "<y2>"
  Bus Selector6/6 -> MATLAB Function/36(z12)  "<z2>"
  Bus Selector/6 -> Bus Selector6/1  "<uva11_12>"
  Bus Selector7/1 -> MATLAB Function/37(x13)  "<x3>"
  Bus Selector7/2 -> MATLAB Function/38(y13)  "<y3>"
  Bus Selector7/3 -> MATLAB Function/39(z13)  "<z3>"
  Bus Selector7/4 -> MATLAB Function/40(x14)  "<x4>"
  Bus Selector7/5 -> MATLAB Function/41(y14)  "<y4>"
  Bus Selector7/6 -> MATLAB Function/42(z14)  "<z4>"
  Bus Selector/7 -> Bus Selector7/1  "<uav13_14>"
  Bus Selector9/1 -> MATLAB Function/43(x15)  "<x5>"
  Bus Selector/10 -> Bus Selector11/1  "<uav19_20>"
  Bus Selector/9 -> Bus Selector10/1  "<uav17_18>"
  Bus Selector9/6 -> MATLAB Function/48(z16)  "<z6>"
  Bus Selector11/1 -> MATLAB Function/55(x19)  "<x9>"
  Bus Selector11/5 -> MATLAB Function/59(y20)  "<y10>"
  Bus Selector10/4 -> MATLAB Function/52(x18)  "<x8>"
  Bus Selector9/3 -> MATLAB Function/45(z15)  "<z5>"
  Bus Selector10/6 -> MATLAB Function/54(z18)  "<z8>"
  Bus Selector10/1 -> MATLAB Function/49(x17)  "<x7>"
  Bus Selector10/2 -> MATLAB Function/50(y17)  "<y7>"
  Bus Selector11/4 -> MATLAB Function/58(x20)  "<x10>"
  Bus Selector11/3 -> MATLAB Function/57(z19)  "<z9>"
  Bus Selector/8 -> Bus Selector9/1  "<uav15_16>"
  Bus Selector9/2 -> MATLAB Function/44(y15)  "<y5>"
  Bus Selector9/5 -> MATLAB Function/47(y16)  "<y6>"
  Bus Selector10/3 -> MATLAB Function/51(z17)  "<z7>"
  Bus Selector10/5 -> MATLAB Function/53(y18)  "<y8>"
  Bus Selector11/2 -> MATLAB Function/56(y19)  "<y9>"
  Bus Selector9/4 -> MATLAB Function/46(x16)  "<x6>"
  Bus Selector11/6 -> MATLAB Function/60(z20)  "<z10>"
  Bus Selector8/4 -> MATLAB Function/64(x22)  "<x2>"
  Bus Selector12/2 -> MATLAB Function/68(y23)  "<y3>"
  Bus Selector8/3 -> MATLAB Function/63(z21)  "<z1>"
  Bus Selector12/5 -> MATLAB Function/71(y24)  "<y4>"
  Bus Selector12/4 -> MATLAB Function/70(x24)  "<x4>"
  Bus Selector8/6 -> MATLAB Function/66(z22)  "<z2>"
  Bus Selector8/1 -> MATLAB Function/61(x21)  "<x1>"
  Bus Selector8/2 -> MATLAB Function/62(y21)  "<y1>"
  Bus Selector/12 -> Bus Selector12/1  "<uav23_24>"
  Bus Selector/11 -> Bus Selector8/1  "<uav21_22>"
  Bus Selector8/5 -> MATLAB Function/65(y22)  "<y2>"
  Bus Selector12/1 -> MATLAB Function/67(x23)  "<x3>"
  Bus Selector12/3 -> MATLAB Function/69(z23)  "<z3>"
  Bus Selector12/6 -> MATLAB Function/72(z24)  "<z4>"

== system SIMULINK_ADP_Tracking/send_ctrl_signal_UAV ==
  uav_ctrl : Inport
  Bus Selector : BusSelector  OutputSignals=ctrl_1_2,ctrl_3_4
  Bus Selector1 : BusSelector  OutputSignals=droneyeeUAV1_states,droneyeeUAV2_states  OutputAsBus=on
  Bus Selector2 : BusSelector  OutputSignals=ctrl_5_6.uav_5,ctrl_5_6.uav_6
  Bus Selector3 : BusSelector  OutputSignals=droneyeeUAV5_states,droneyeeUAV6_states
  Bus Selector4 : BusSelector  OutputSignals=ctrl_9_10.uav_9,ctrl_9_10.uav_10
  Bus Selector5 : BusSelector  OutputSignals=droneyeeUAV9_states,droneyeeUAV10_states
  Bus Selector6 : BusSelector  OutputSignals=droneyeeUAV3_states,droneyeeUAV4_states  OutputAsBus=on
  Bus Selector7 : BusSelector  OutputSignals=droneyeeUAV7_states,droneyeeUAV8_states
  Bus Selector8 : BusSelector  OutputSignals=ctrl_7_8.uav_7,ctrl_7_8.uav_8
  Send Command 1 : Subsystem
  Send Command 10 : Subsystem
  Send Command 2 : Subsystem
  Send Command 3 : Subsystem
  Send Command 4 : Subsystem
  Send Command 5 : Subsystem
  Send Command 6 : Subsystem
  Send Command 7 : Subsystem
  Send Command 8 : Subsystem
  Send Command 9 : Subsystem
  Subsystem : Subsystem
  To Workspace : ToWorkspace  VariableName=simout  SaveFormat=Structure With Time  SampleTime=-1
  wires:
  Bus Selector/1 -> Send Command 2/2(u), Send Command 1/2(u)  "<ctrl_1_2>"
  Bus Selector1/1 -> Send Command 2/1(pos), Send Command 1/1(pos)
  Bus Selector/2 -> Send Command 3/2(u), Send Command 4/2(u)  "<ctrl_3_4>"
  Bus Selector2/1 -> Send Command 5/2(u)  "<uav_5>"
  Bus Selector3/1 -> Send Command 5/1(pos)  "<droneyeeUAV5_states>"
  Bus Selector5/1 -> Send Command 9/1(pos)  "<droneyeeUAV9_states>"
  Bus Selector4/1 -> Send Command 9/2(u)  "<uav_9>"
  [uav_states] -> Bus Selector1/1
  Bus Selector6/1 -> Send Command 4/1(pos), Send Command 3/1(pos)
  [uav_states] -> Bus Selector3/1
  [uav_states] -> Bus Selector5/1
  uav_ctrl/1 -> Bus Selector8/1, To Workspace/1, Subsystem/2(ctrl), Bus Selector4/1, Bus Selector2/1, Bus Selector/1
  [uav_states] -> Bus Selector6/1
  [uav1_24_d] -> Subsystem/1(states_d)
  [uav_states] -> Bus Selector7/1
  Bus Selector7/1 -> Send Command 7/1(pos)  "<droneyeeUAV7_states>"
  Bus Selector7/2 -> Send Command 8/1(pos)  "<droneyeeUAV8_states>"
  Bus Selector8/2 -> Send Command 8/2(u)  "<uav_8>"
  Bus Selector8/1 -> Send Command 7/2(u)  "<uav_7>"
  Bus Selector3/2 -> Send Command 6/1(pos)  "<droneyeeUAV6_states>"
  Bus Selector2/2 -> Send Command 6/2(u)  "<uav_6>"
  Bus Selector5/2 -> Send Command 10/1(pos)  "<droneyeeUAV10_states>"
  Bus Selector4/2 -> Send Command 10/2(u)  "<uav_10>"

== system SIMULINK_ADP_Tracking/send_ctrl_signal_car1 ==
  uav_ctrl : Inport
  Bus Selector : BusSelector  OutputSignals=ctrlCAR1_2,ctrlCAR3_4
  Bus Selector1 : BusSelector  OutputSignals=droneyeeCAR1_states,droneyeeCAR2_states  OutputAsBus=on
  Bus Selector2 : BusSelector  OutputSignals=ctrlCAR5_6.CAR5,ctrlCAR5_6.CAR6
  Bus Selector3 : BusSelector  OutputSignals=droneyeeCAR5_states,droneyeeCAR6_states
  Bus Selector4 : BusSelector  OutputSignals=ctrlCAR9_10.CAR9,ctrlCAR9_10.CAR10
  Bus Selector5 : BusSelector  OutputSignals=droneyeeCAR9_states,droneyeeCAR10_states
  Bus Selector6 : BusSelector  OutputSignals=droneyeeCAR3_states,droneyeeCAR4_states  OutputAsBus=on
  Bus Selector7 : BusSelector  OutputSignals=droneyeeCAR7_states,droneyeeCAR8_states
  Bus Selector8 : BusSelector  OutputSignals=ctrlCAR7_8.CAR7,ctrlCAR7_8.CAR8
  Send Command 1 : Subsystem
  Send Command 10 : Subsystem
  Send Command 2 : Subsystem
  Send Command 3 : Subsystem
  Send Command 4 : Subsystem
  Send Command 5 : Subsystem
  Send Command 6 : Subsystem
  Send Command 7 : Subsystem
  Send Command 8 : Subsystem
  Send Command 9 : Subsystem
  Subsystem : Subsystem
  To Workspace : ToWorkspace  VariableName=simoutcar  SaveFormat=Structure With Time  SampleTime=-1
  wires:
  Bus Selector/1 -> Send Command 2/2(u), Send Command 1/2(u)  "<ctrlCAR1_2>"
  Bus Selector1/1 -> Send Command 2/1(pos), Send Command 1/1(pos)
  Bus Selector/2 -> Send Command 3/2(u), Send Command 4/2(u)  "<ctrlCAR3_4>"
  Bus Selector2/1 -> Send Command 5/2(u)  "<CAR5>"
  Bus Selector3/1 -> Send Command 5/1(pos)  "<droneyeeCAR5_states>"
  Bus Selector5/1 -> Send Command 9/1(pos)  "<droneyeeCAR9_states>"
  Bus Selector4/1 -> Send Command 9/2(u)  "<CAR9>"
  [uav_states] -> Bus Selector1/1
  Bus Selector6/1 -> Send Command 4/1(pos), Send Command 3/1(pos)
  [uav_states] -> Bus Selector3/1
  [uav_states] -> Bus Selector5/1
  uav_ctrl/1 -> Bus Selector8/1, To Workspace/1, Subsystem/2(ctrl), Bus Selector4/1, Bus Selector2/1, Bus Selector/1
  [uav_states] -> Bus Selector6/1
  [car1_10_d] -> Subsystem/1(states_d)
  [uav_states] -> Bus Selector7/1
  Bus Selector7/1 -> Send Command 7/1(pos)  "<droneyeeCAR7_states>"
  Bus Selector7/2 -> Send Command 8/1(pos)  "<droneyeeCAR8_states>"
  Bus Selector8/2 -> Send Command 8/2(u)  "<CAR8>"
  Bus Selector8/1 -> Send Command 7/2(u)  "<CAR7>"
  Bus Selector3/2 -> Send Command 6/1(pos)  "<droneyeeCAR6_states>"
  Bus Selector2/2 -> Send Command 6/2(u)  "<CAR6>"
  Bus Selector5/2 -> Send Command 10/1(pos)  "<droneyeeCAR10_states>"
  Bus Selector4/2 -> Send Command 10/2(u)  "<CAR10>"
